simulink model "TestAirData"  (R2016b)
settings: Solver=VariableStepAuto  StartTime=0.0  StopTime=10.0  RelTol=1e-3
model workspace (MAT data in the model file):
  sens = Simulink.Parameter
  sens.Value.rAirData_S_m = [0.0254; 0.3556; 0]
  sens.Value.rAirData_SB_m = [-0.0254; 0.3556; 0]
  sens.Value.sAirData_SB_rad = [0; 0; 0]
  sens.Value.T_B2AirData = [1  0  0; 0  1  0; 0  0  1]
  sens.Value.errEnable = 1
  sens.Value.PdTF_num = 2199.11485751
  sens.Value.PdTF_den = [1 2199.11485751]
  sens.Value.tempTF_num = 2199.11485751
  sens.Value.tempTF_den = [1 2199.11485751]
  sens.Value.PdTimeDelay_s = 1e-05
  sens.Value.tempTimeDelay_s = 1e-05
  sens.Value.PdScf = 1
  sens.Value.PdBias = 0
  sens.Value.PdSigma = 60
  sens.Value.PdSeed = 14377
  sens.Value.tempScf = 1
  sens.Value.tempBias = 0
  sens.Value.tempSigma = 0.5
  sens.Value.tempSeed = 26057
  sens.Value.PsTF_num = 2199.11485751
  sens.Value.PsTF_den = [1 2199.11485751]
  sens.Value.PsTimeDelay_s = 1e-05
  sens.Value.PsScf = 1
  sens.Value.PsBias = 0
  sens.Value.PsSigma = 750
  sens.Value.PsSeed = 25084
  sens.Value.tubeLength_m = 0.5
  sens.Value.vSound_mps = 340
  sens.Value.tubeTF_num = 1140926.26877
  sens.Value.tubeTF_den = [1 640.884901332 1140926.26877]
  sens.Value.timeSample_s = 0.02
  sens.DataType = 'struct'
  sens.Dimensions = [1 1]
libraries: Sensors_Lib x4
settings Model: ParameterArgumentNames=sens  Creator=katiekwiz  LastModifiedBy=katiekwiz

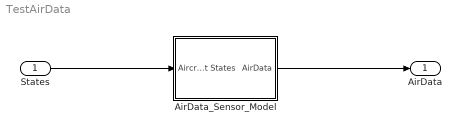
== system TestAirData ==
  States : Inport
  AirData_Sensor_Model : Subsystem  Variant=on  VariantControl=Variant1
  AirData : Outport
  wires:
  States/1 -> AirData_Sensor_Model/1("Aircraft States ")
  AirData_Sensor_Model/1(" AirData") -> AirData/1

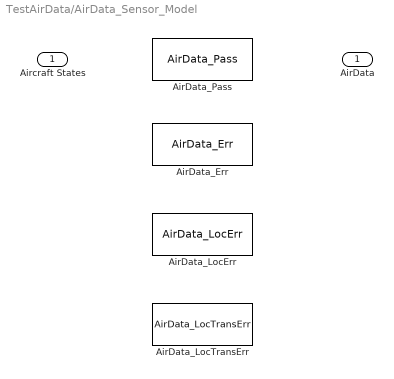
== system TestAirData/AirData_Sensor_Model ==
  "Aircraft States " : Inport
  AirData_Err : Sensors_Lib/AirData Sensor Models/AirData_Err  VariantControl=VarAirData_Err
      settings: AttributesFormatString=Variant: %<VariantControl> : %<Variant>
  AirData_LocErr : Sensors_Lib/AirData Sensor Models/AirData_LocErr  VariantControl=VarAirData_LocErr
      settings: AttributesFormatString=Variant: %<VariantControl> : %<Variant>
  AirData_LocTransErr : Sensors_Lib/AirData Sensor Models/AirData_LocTransErr  VariantControl=VarAirData_LocTransErr
      settings: AttributesFormatString=Variant: %<VariantControl> : %<Variant>
  AirData_Pass : Sensors_Lib/AirData Sensor Models/AirData_Pass  VariantControl=VarAirData_Pass
      settings: AttributesFormatString=Variant: %<VariantControl> : %<Variant>
  " AirData" : Outport
